simulink model "Calculator"  (R2016a)
settings: Solver=FixedStepDiscrete  StartTime=0.0  StopTime=10.0  RelTol=1e-3
settings Model: Creator=Muhammed  LastModifiedBy=Muhammed
settings OptimizationCC: DefaultParameterBehavior=Inlined  InlineInvariantSignals=on  EnableMemcpy=off  OptimizeModelRefInitCode=on  LifeSpan=1
settings DebuggingCC: UnderspecifiedInitializationDetection=Classic  MergeDetectMultiDrivingBlocksExec=none
settings ModelReferenceCC: PropagateSignalLabelsOutOfModel=off
settings RTWCC: SystemTargetFile=ert.tlc  GenCodeOnly=on  TemplateMakefile=ert_default_tmf  GenerateReport=on  IncludeHyperlinkInReport=on  LaunchReport=on  GenerateTraceInfo=on  GenerateTraceReport=on  GenerateTraceReportSl=on  GenerateTraceReportSf=on  GenerateTraceReportEml=on
settings CodeAppCC: ForceParamTrailComments=on  IgnoreCustomStorageClasses=off  OperatorAnnotations=on  SimulinkDataObjDesc=on  SFDataObjDesc=on  MATLABFcnDesc=on  InsertBlockDesc=on  MATLABSourceComments=on
settings ERTTargetCC: GenerateSampleERTMain=on  InlinedParameterPlacement=NonHierarchical  ERTCustomFileTemplate=example_file_process.tlc

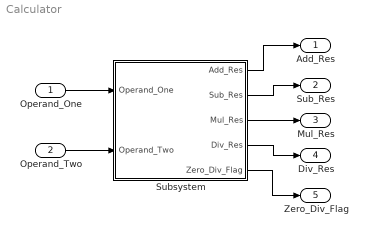
== system Calculator ==
  Operand_One : Inport
  Operand_Two : Inport  Port=2
  Subsystem : Subsystem  TreatAsAtomicUnit=on
      settings: MinAlgLoopOccurrences=on  RTWFcnNameOpts=Use subsystem name
  Add_Res : Outport
  Sub_Res : Outport  Port=2
  Mul_Res : Outport  Port=3
  "Div_Res " : Outport  Port=4
  Zero_Div_Flag : Outport  Port=5
  wires:
  Operand_One/1 -> Subsystem/1(Operand_One)
  Operand_Two/1 -> Subsystem/2(Operand_Two)
  Subsystem/1(Add_Res) -> Add_Res/1
  Subsystem/2(Sub_Res) -> Sub_Res/1
  Subsystem/3(Mul_Res) -> Mul_Res/1
  Subsystem/4("Div_Res ") -> "Div_Res "/1
  Subsystem/5(Zero_Div_Flag) -> Zero_Div_Flag/1

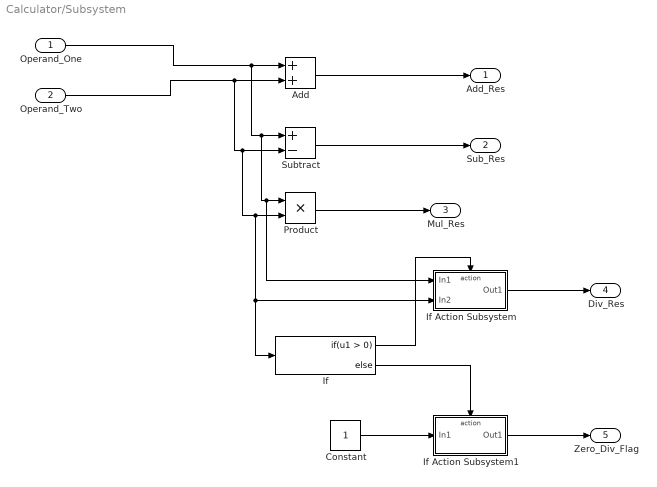
== system Calculator/Subsystem ==
  Operand_One : Inport
  Operand_Two : Inport  Port=2
  Add : Sum
  Constant : Constant
  If : If
  If Action Subsystem : Subsystem  TreatAsAtomicUnit=on
  If Action Subsystem1 : Subsystem  TreatAsAtomicUnit=on
  Product : Product
  Subtract : Sum  Inputs=+-
  Add_Res : Outport
  Sub_Res : Outport  Port=2
  Mul_Res : Outport  Port=3
  "Div_Res " : Outport  Port=4
  Zero_Div_Flag : Outport  Port=5
  wires:
  Product/1 -> Mul_Res/1
  Operand_Two/1 -> If Action Subsystem/2(In2), If/1, Product/2, Subtract/2, Add/2
  Add/1 -> Add_Res/1
  Subtract/1 -> Sub_Res/1
  If Action Subsystem/1(Out1) -> "Div_Res "/1
  Constant/1 -> If Action Subsystem1/1(In1)
  If/2 -> If Action Subsystem1/Action
  Operand_One/1 -> If Action Subsystem/1(In1), Product/1, Subtract/1, Add/1
  If Action Subsystem1/1(Out1) -> Zero_Div_Flag/1
  If/1 -> If Action Subsystem/Action

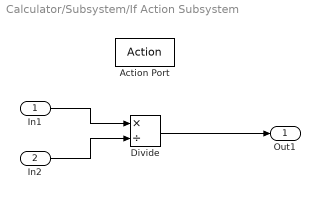
== system Calculator/Subsystem/If Action Subsystem ==
  In1 : Inport
  In2 : Inport  Port=2
  Action Port : ActionPort  ActionType=then
  Divide : Product  Inputs=*/
  Out1 : Outport
  wires:
  In1/1 -> Divide/1
  In2/1 -> Divide/2
  Divide/1 -> Out1/1

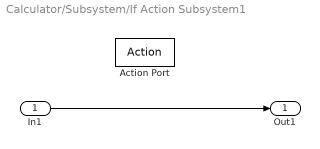
== system Calculator/Subsystem/If Action Subsystem1 ==
  In1 : Inport
  Action Port : ActionPort  ActionType=else
  Out1 : Outport
  wires:
  In1/1 -> Out1/1
